simulink model "afm_tracker"  (R2016b)
settings: Solver=VariableStepAuto  StartTime=0.0  StopTime=trun  RelTol=1e-3
values from neighbouring files (symbols this model uses):
  D_x = ss(tf([1 0]*Ki_x, [1 -1], Ts))    [mu_path.m]    (also in mu_spectrum.m = ss(tf([1]*Ki_x, [1 -1], Ts)))
  D_y = D_x    [mu_path.m]
  M = 11    [mu_path.m]
  mu2volts = 1/5    (= 0.2)    [mu_path.m]    (also in mu_spectrum.m; setup_rasterscan.m; setup_rasterscan_singleperiod.m)
libraries: cstblocks x5
settings Model: Creator=arnold  LastModifiedBy=arnold

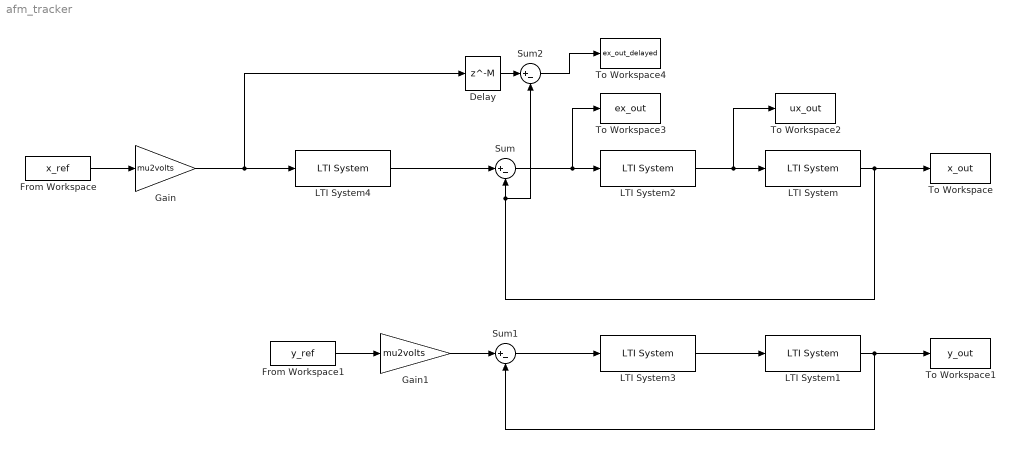
== system afm_tracker ==
  Delay : Delay  DelayLength=M
  From Workspace : FromWorkspace  VariableName=x_ref  SampleTime=0
  From Workspace1 : FromWorkspace  VariableName=y_ref  SampleTime=0
  Gain : Gain  Gain=mu2volts
  Gain1 : Gain  Gain=mu2volts
  LTI System : cstblocks/LTI System  sys=G_x  IC=x0
  LTI System1 : cstblocks/LTI System  sys=G_y  IC=y0
  LTI System2 : cstblocks/LTI System  sys=ss(D_x)  IC=Dx_0
  LTI System3 : cstblocks/LTI System  sys=ss(D_y)  IC=Dy_0
  LTI System4 : cstblocks/LTI System  sys=FFCLI_x  IC=Dx_0
  Sum : Sum  Inputs=|+-
  Sum1 : Sum  Inputs=|+-
  Sum2 : Sum  Inputs=|+-
  To Workspace : ToWorkspace  VariableName=x_out  SaveFormat=Timeseries  SampleTime=-1
  To Workspace1 : ToWorkspace  VariableName=y_out  SaveFormat=Timeseries  SampleTime=-1
  To Workspace2 : ToWorkspace  VariableName=ux_out  SaveFormat=Timeseries  SampleTime=-1
  To Workspace3 : ToWorkspace  VariableName=ex_out  SaveFormat=Timeseries  SampleTime=-1
  To Workspace4 : ToWorkspace  VariableName=ex_out_delayed  SaveFormat=Timeseries  SampleTime=-1
  wires:
  Sum/1 -> To Workspace3/1, LTI System2/1
  LTI System/1 -> To Workspace/1, Sum2/2, Sum/2
  LTI System2/1 -> To Workspace2/1, LTI System/1
  Sum1/1 -> LTI System3/1
  LTI System1/1 -> To Workspace1/1, Sum1/2
  LTI System3/1 -> LTI System1/1
  From Workspace/1 -> Gain/1
  Gain1/1 -> Sum1/1
  From Workspace1/1 -> Gain1/1
  Delay/1 -> Sum2/1
  Sum2/1 -> To Workspace4/1
  LTI System4/1 -> Sum/1
  Gain/1 -> Delay/1, LTI System4/1
